simulink model "projet_ABS_last"  (R2022b)
settings: Solver=VariableStepAuto  StartTime=0.0  StopTime=17  RelTol=1e-3
InitFcn:
  | ABS_config
values from neighbouring files (symbols this model uses):
  f0 = 0.8    [ABS_config.m]
  J = 0.5    [ABS_config.m]
  m = 1000    [ABS_config.m]
  N = m*g/4    (= 2452.5)    [ABS_config.m]
  r_roue = 0.3    [ABS_config.m]
  v0 = 100    [ABS_config.m]
libraries: simulink x2
settings Model: Creator=GEII Robot  LastModifiedBy=abenguet600
settings SolverCC: AlgebraicLoopSolver=TrustRegion
settings DataIOCC: ReturnWorkspaceOutputs=off
settings DebuggingCC: UnconnectedInputMsg=warning  UnconnectedOutputMsg=warning  UnconnectedLineMsg=warning  SFMachineParentedDataDiag=warning  ArithmeticOperatorsInVariantConditions=warning
settings ModelReferenceCC: EnableRefExpFcnMdlSchedulingChecks=on
settings SFSimCC: SimUseLocalCustomCode=off  CustomCodeUndefinedFunction=UseInterfaceOnly
settings RTWCC: RTWUseLocalCustomCode=off

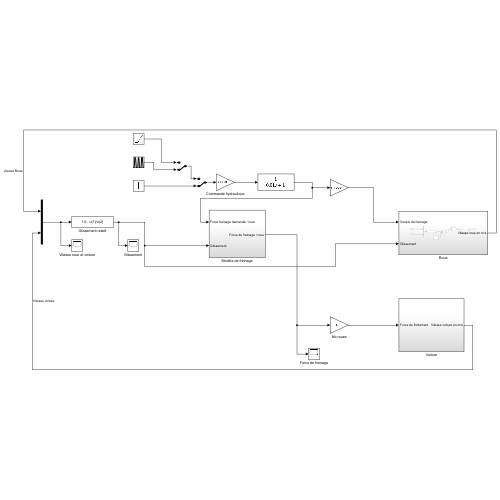
[thumbnail: Simulink's stored preview of the top-level diagram]
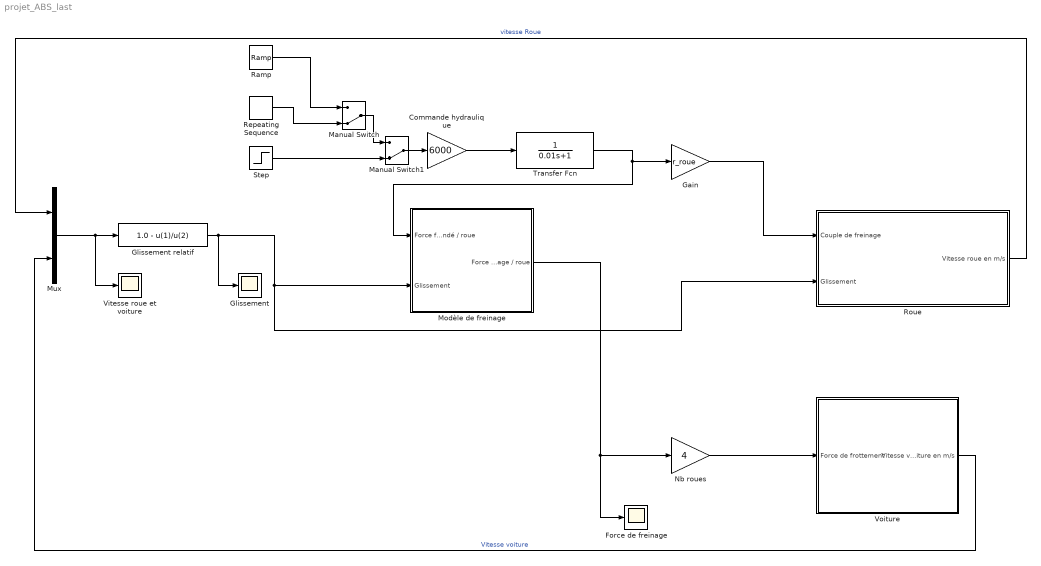
== system projet_ABS_last ==
  Commande hydraulique : Gain  Gain=6000
  Force de freinage : Scope
  Gain : Gain  Gain=r_roue
  Glissement : Scope
  Glissement relatif : Fcn  Expr=1.0 - u(1)/u(2)
  Manual Switch : ManualSwitch  CurrentSetting=0
  Manual Switch1 : ManualSwitch  CurrentSetting=0
  Modèle de freinage : Subsystem
  Mux : Mux  Inputs=2
  Nb roues : Gain  Gain=4
  Ramp : simulink/Sources/Ramp  slope=1  start=5  InitialOutput=0
  Repeating Sequence : simulink/Sources/Repeating Sequence  rep_seq_t=[0 10 20 30 40 50]  rep_seq_y=[0 0 1 1 0 0]
  Roue : Subsystem
  Step : Step  Time=5  SampleTime=0
  Transfer Fcn : TransferFcn  Denominator=[0.01 1]
  Vitesse roue et voiture : Scope
  Voiture : Subsystem
  wires:
  Glissement relatif/1 -> Glissement/1, Roue/2(Glissement), Modèle de freinage/2(Glissement)
  Modèle de freinage/1(Force de freinage / roue) -> Force de freinage/1, Nb roues/1
  Gain/1 -> Roue/1(Couple de freinage)
  Nb roues/1 -> Voiture/1(Force de frottement)
  Mux/1 -> Vitesse roue et voiture/1, Glissement relatif/1
  Voiture/1(Vitesse voiture en m/s) -> Mux/2  "Vitesse voiture"
  Roue/1(Vitesse roue en m/s) -> Mux/1  "vitesse Roue"
  Manual Switch/1 -> Manual Switch1/1
  Manual Switch1/1 -> Commande hydraulique/1
  Ramp/1 -> Manual Switch/1
  Repeating Sequence/1 -> Manual Switch/2
  Step/1 -> Manual Switch1/2
  Commande hydraulique/1 -> Transfer Fcn/1
  Transfer Fcn/1 -> Modèle de freinage/1(Force freinage demandé / roue), Gain/1

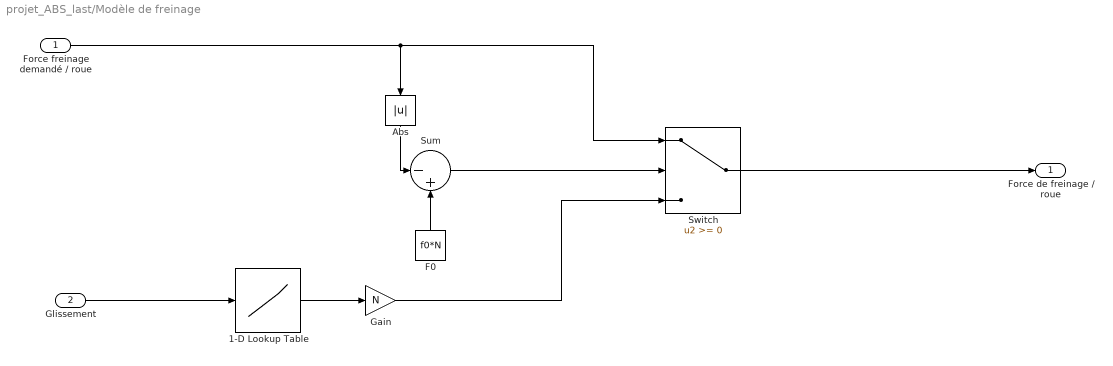
== system projet_ABS_last/Modèle de freinage ==
  Force freinage demandé / roue : Inport
  Glissement : Inport  Port=2
  1-D Lookup Table : Lookup_n-D  NumberOfTableDimensions=1  BreakpointsForDimension1=[0,0.025,0.05,0.1,0.15,0.2,0.25,0.3,0.35,0.4,0.45,0.5,0.55,0.6,0.65,0.7,0.75,0.8,0.85,0.9,0.95,1]  Table=[0,0.34,0.6,0.86,0.91,0.86,0.83,0.76,0.72,0.71,0.7,0.68,0.67,0.66,0.65,0.64,0.63,0.63,0.62,0.615,0.61,0.61]  InternalRulePriority=Speed  RndMeth=Simplest
  Abs : Abs  SaturateOnIntegerOverflow=off
  F0 : Constant  Value=f0*N
  Gain : Gain  Gain=N
  Sum : Sum  Inputs=|-+
  Switch : Switch  SaturateOnIntegerOverflow=off  InputSameDT=off
  Force de freinage / roue : Outport  VectorParamsAs1DForOutWhenUnconnected=off
  wires:
  Glissement/1 -> 1-D Lookup Table/1
  Force freinage demandé / roue/1 -> Abs/1, Switch/1
  1-D Lookup Table/1 -> Gain/1
  Switch/1 -> Force de freinage / roue/1
  Gain/1 -> Switch/3
  Sum/1 -> Switch/2
  F0/1 -> Sum/2
  Abs/1 -> Sum/1

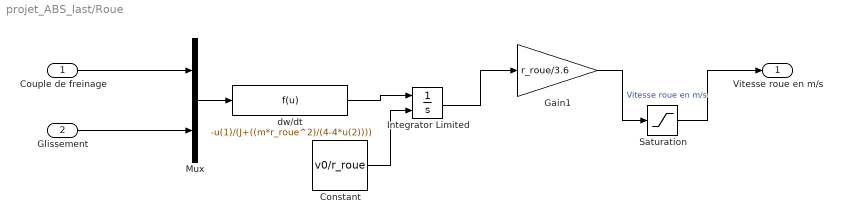
== system projet_ABS_last/Roue ==
  Couple de freinage : Inport
  Glissement : Inport  Port=2
  Constant : Constant  Value=v0/r_roue
  Gain1 : Gain  Gain=r_roue/3.6
  Integrator Limited : Integrator  InitialConditionSource=external  LimitOutput=on  UpperSaturationLimit=1000  LowerSaturationLimit=0
  Mux : Mux  Inputs=2
  Saturation : Saturate  UpperLimit=1000  LowerLimit=0
  dw/dt : Fcn  Expr=-u(1)/(J+((m*r_roue^2)/(4-4*u(2))))
  Vitesse roue en m/s : Outport
  wires:
  Gain1/1 -> Saturation/1  "Vitesse roue en m/s"
  Couple de freinage/1 -> Mux/1
  Glissement/1 -> Mux/2
  Mux/1 -> dw/dt/1
  dw/dt/1 -> Integrator Limited/1
  Integrator Limited/1 -> Gain1/1
  Constant/1 -> Integrator Limited/2
  Saturation/1 -> Vitesse roue en m/s/1

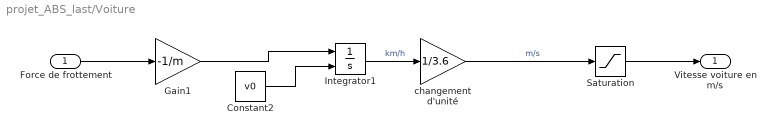
== system projet_ABS_last/Voiture ==
  Force de frottement : Inport
  Constant2 : Constant  Value=v0
  Gain1 : Gain  Gain=-1/m
  Integrator1 : Integrator  InitialConditionSource=external
  Saturation : Saturate  UpperLimit=1000  LowerLimit=0
  changement d'unité : Gain  Gain=1/3.6
  Vitesse voiture en m/s : Outport  VectorParamsAs1DForOutWhenUnconnected=off
  wires:
  Gain1/1 -> Integrator1/1
  Constant2/1 -> Integrator1/2
  Integrator1/1 -> changement d'unité/1  "km/h"
  Force de frottement/1 -> Gain1/1
  changement d'unité/1 -> Saturation/1  "m/s"
  Saturation/1 -> Vitesse voiture en m/s/1
